simulink model "W09_2_qos_test"  (R2024b)
settings: Solver=FixedStepDiscrete  StartTime=0.0  StopTime=T_end  FixedStep=Ts  RelTol=1e-3
values from neighbouring files (symbols this model uses):
  Ts = 0.005    [W04_setup.m]    (also in W09_offline_run.m = evalin('base','Ts'); W09_setup.m)
libraries: ros2lib x2
settings Model: Creator=admin  LastModifiedBy=admin

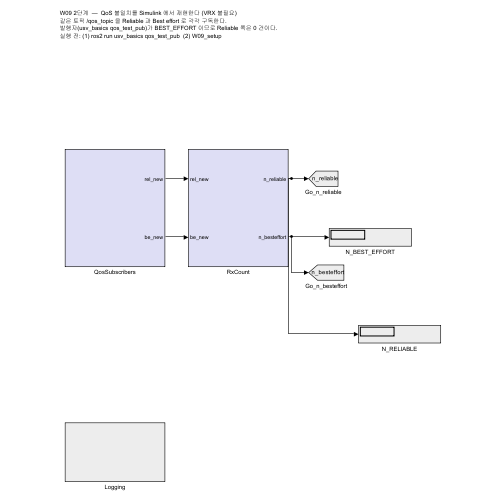
[thumbnail: Simulink's stored preview of the top-level diagram]
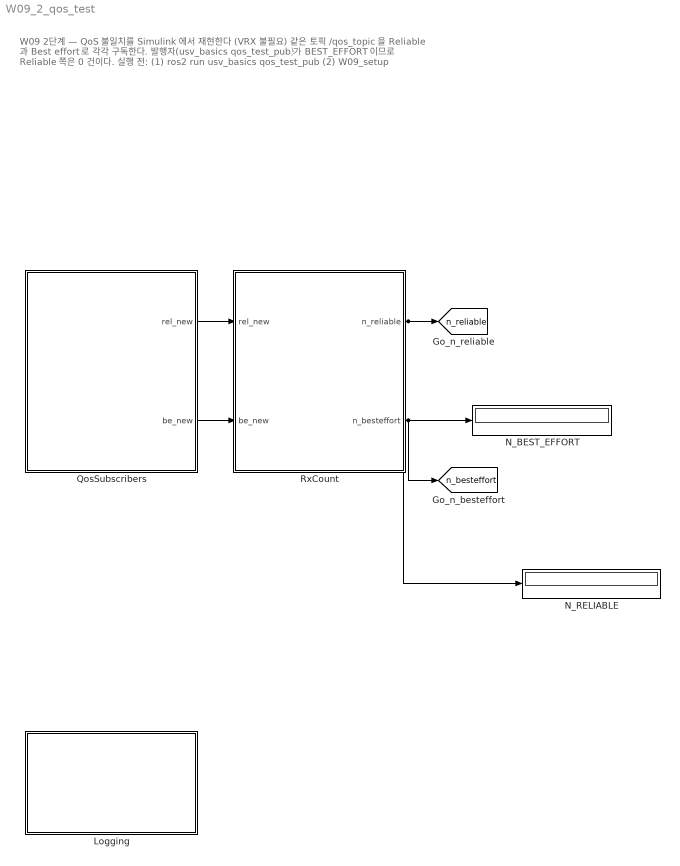
== system W09_2_qos_test ==
  note: W09 2단계  —  QoS 불일치를 Simulink 에서 재현한다 (VRX 불필요)
      | 같은 토픽 /qos_topic 을 Reliable 과 Best effort 로 각각 구독한다.
      | 발행자(usv_basics qos_test_pub)가 BEST_EFFORT 이므로 Reliable 쪽은 0 건이다.
      | 실행 전: (1) ros2 run usv_basics qos_test_pub  (2) W09_setup
  Logging : Subsystem
  N_BEST_EFFORT : Display
  N_RELIABLE : Display
  QosSubscribers : Subsystem
  RxCount : Subsystem
  tag scope: n_besteffort=global, n_reliable=global
  wires:
  QosSubscribers/1(rel_new) -> RxCount/1(rel_new)
  QosSubscribers/2(be_new) -> RxCount/2(be_new)
  RxCount/2(n_besteffort) -> N_BEST_EFFORT/1, [n_besteffort]
  RxCount/1(n_reliable) -> N_RELIABLE/1, [n_reliable]

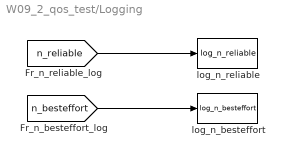
== system W09_2_qos_test/Logging ==
  log_n_besteffort : ToWorkspace  VariableName=log_n_besteffort  SaveFormat=Timeseries  SampleTime=Ts
  log_n_reliable : ToWorkspace  VariableName=log_n_reliable  SaveFormat=Timeseries  SampleTime=Ts
  wires:
  [n_reliable] -> log_n_reliable/1
  [n_besteffort] -> log_n_besteffort/1

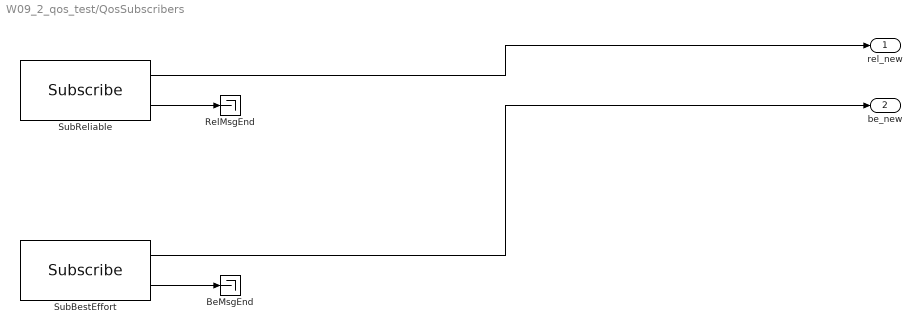
== system W09_2_qos_test/QosSubscribers ==
  BeMsgEnd : Terminator
  RelMsgEnd : Terminator
  SubBestEffort : ros2lib/Subscribe  topicSource=Specify your own  topic=/qos_topic  messageType=std_msgs/String  sampleTime=Ts  QOSHistory=Keep last  QOSDepth=1  QOSReliability=Best effort  QOSDurability=Volatile  QOSDeadline=Inf  QOSLifespan=Inf  QOSLiveliness=Automatic  QOSLeaseDuration=Inf  QOSAvoidROSNamespaceConventions=off
  SubReliable : ros2lib/Subscribe  topicSource=Specify your own  topic=/qos_topic  messageType=std_msgs/String  sampleTime=Ts  QOSHistory=Keep last  QOSDepth=1  QOSReliability=Reliable  QOSDurability=Volatile  QOSDeadline=Inf  QOSLifespan=Inf  QOSLiveliness=Automatic  QOSLeaseDuration=Inf  QOSAvoidROSNamespaceConventions=off
  rel_new : Outport
  be_new : Outport  Port=2
  wires:
  SubReliable/2 -> RelMsgEnd/1
  SubBestEffort/2 -> BeMsgEnd/1
  SubReliable/1 -> rel_new/1
  SubBestEffort/1 -> be_new/1

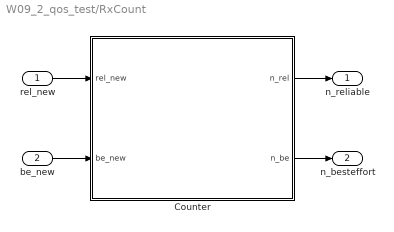
== system W09_2_qos_test/RxCount ==
  rel_new : Inport
  be_new : Inport  Port=2
  Counter : MATLAB Function  TreatAsAtomicUnit=on
  n_reliable : Outport
  n_besteffort : Outport  Port=2
  wires:
  be_new/1 -> Counter/2(be_new)
  rel_new/1 -> Counter/1(rel_new)
  Counter/1(n_rel) -> n_reliable/1
  Counter/2(n_be) -> n_besteffort/1

== matlab function W09_2_qos_test/RxCount/Counter ==
  data: rel_new input; n_rel output; be_new input; n_be output
function [n_rel, n_be] = Counter(rel_new, be_new)
%#codegen
% Count messages received by each subscriber.
% Publisher (qos_test_pub) is BEST_EFFORT, so a RELIABLE subscriber
% is incompatible and receives nothing at all.
persistent nr nb
if isempty(nr), nr = 0; nb = 0; end
if rel_new, nr = nr + 1; end
if be_new,  nb = nb + 1; end
n_rel = nr;  n_be = nb;
